simulink model "multirotor_simple_takeoff"  (R2023b)
settings: Solver=VariableStepAuto  StartTime=0.0  StopTime=10.0  RelTol=1e-3
libraries: robotcorelib x1, sensorgpslib x1, uavalgslib x1, uavutilslib x1
settings Model: Creator=rakshan  LastModifiedBy=rakshan
settings DebuggingCC: ParameterPrecisionLossMsg=none

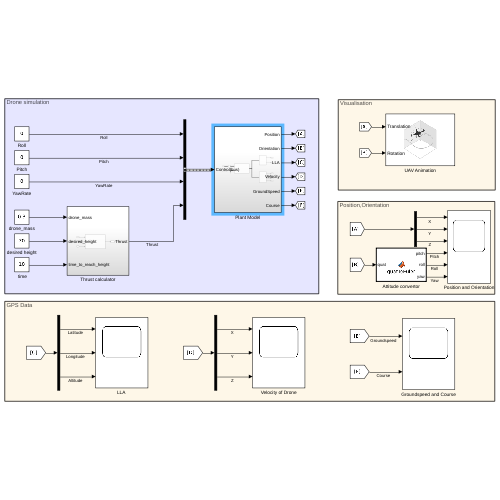
[thumbnail: Simulink's stored preview of the top-level diagram]
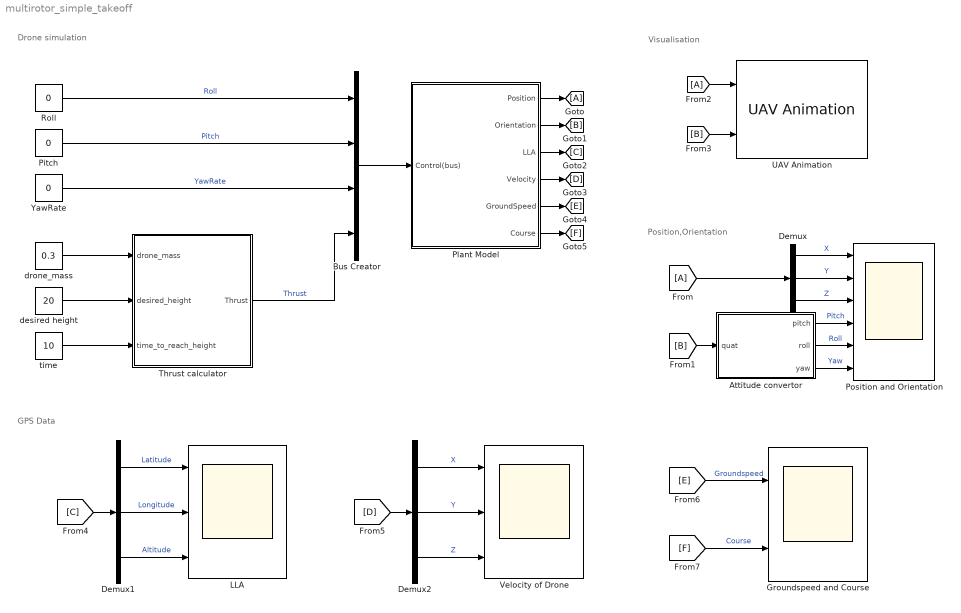
== system multirotor_simple_takeoff ==
  note: GPS Data
  note: Position,Orientation
  note: Visualisation
  note: Drone simulation
  " time" : Constant  Value=10
  Attitude convertor : MATLAB Function  TreatAsAtomicUnit=on
  Bus Creator : BusCreator  Inputs=4  OutDataTypeStr=Bus: uavGuidanceControlBus  NonVirtualBus=on
      settings: InheritFromInputs=off
  Demux : Demux  Outputs=3
  Demux1 : Demux  Outputs=3
  Demux2 : Demux  Outputs=3
  From : From
  From2 : From
  Goto : Goto
  Groundspeed and Course : Scope  NumInputPorts=2
  "LLA " : Scope  NumInputPorts=3
  Pitch : Constant  Value=0  OutDataTypeStr=single
  Plant Model : Subsystem
  Position and Orientation : Scope  NumInputPorts=6
  Roll : Constant  Value=0  OutDataTypeStr=single
  Thrust calculator : Subsystem
  UAV Animation : uavutilslib/UAV Animation  UAVType=Multirotor  UAVSize=3  InertialZDirection=Down  SampleTime=-1
  Velocity of Drone : Scope  NumInputPorts=3
  YawRate : Constant  Value=0  OutDataTypeStr=single
  desired height : Constant  Value=20
  drone_mass : Constant  Value=0.3
  wires:
  Roll/1 -> Bus Creator/1  "Roll"
  Pitch/1 -> Bus Creator/2  "Pitch"
  YawRate/1 -> Bus Creator/3  "YawRate"
  drone_mass/1 -> Thrust calculator/1(drone_mass)
  desired height/1 -> Thrust calculator/2(desired_height)
  " time"/1 -> Thrust calculator/3(time_to_reach_height)
  Thrust calculator/1(Thrust) -> Bus Creator/4  "Thrust"
  Bus Creator/1 -> Plant Model/1(Control(bus))
  Plant Model/1(Position) -> Goto/1
  Plant Model/2(Orientation) -> [B]
  Demux/2 -> Position and Orientation/2  "Y"
  Demux/3 -> Position and Orientation/3  "Z"
  Demux/1 -> Position and Orientation/1  "X"
  Attitude convertor/1(pitch) -> Position and Orientation/4  "Pitch"
  Attitude convertor/2(roll) -> Position and Orientation/5  "Roll"
  Attitude convertor/3(yaw) -> Position and Orientation/6  "Yaw"
  From/1 -> Demux/1
  [B] -> Attitude convertor/1(quat)
  Plant Model/3(LLA) -> [C]
  Plant Model/4(Velocity) -> [D]
  Plant Model/5(GroundSpeed) -> [E]
  Plant Model/6(Course) -> [F]
  From2/1 -> UAV Animation/1
  [B] -> UAV Animation/2
  Demux1/2 -> "LLA "/2  "Longitude"
  Demux1/1 -> "LLA "/1  "Latitude"
  Demux1/3 -> "LLA "/3  "Altitude"
  [C] -> Demux1/1
  Demux2/2 -> Velocity of Drone/2  "Y"
  Demux2/3 -> Velocity of Drone/3  "Z"
  [D] -> Demux2/1
  Demux2/1 -> Velocity of Drone/1  "X"
  [E] -> Groundspeed and Course/1  "Groundspeed"
  [F] -> Groundspeed and Course/2  "Course"

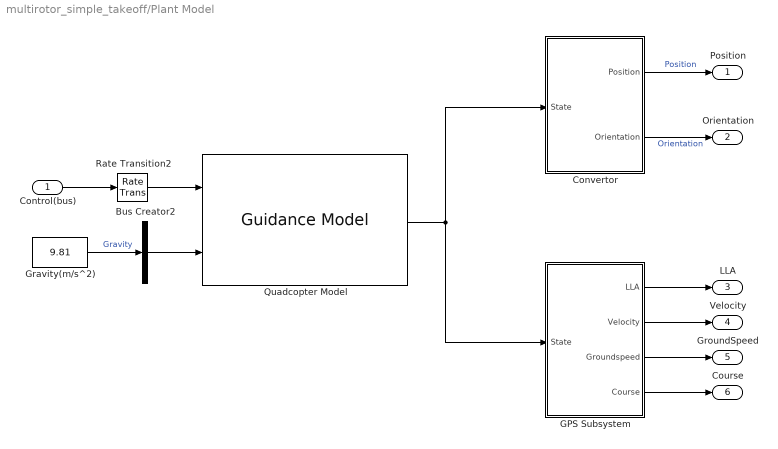
== system multirotor_simple_takeoff/Plant Model ==
  Control(bus) : Inport
  Bus Creator2 : BusCreator  Inputs=1  OutDataTypeStr=Bus: uavGuidanceEnvironmentBus  NonVirtualBus=on
  Convertor : Subsystem
  GPS Subsystem : Subsystem
  Gravity(m/s^2) : Constant  Value=9.81  OutDataTypeStr=single
  Quadcopter Model : uavalgslib/Guidance Model  ModelType=MultirotorGuidance  SpecifiedDataType=single  SimulateUsing=Code generation  InitialWorldPositionMultirotor=[0; 0; 0]  InitialWorldVelocityMultirotor=[0; 0; 0]  InitialEulerZYXMultirotor=[0; 0; 0]  InitialBodyAngularRateRPYMultirotor=[0; 0; 0]  InitialThrustMultirotor=0  InitialNorthFixedWing=0  InitialEastFixedWing=0  InitialHeightFixedWing=0  InitialAirSpeedFixedWing=0  InitialHeadingAngleFixedWing=0  InitialFlightPathAngleFixedWing=0  InitialRollAngleFixedWing=0  InitialRollAngleRateFixedWing=0  PDRollMultirotor=[3402.97,116.67]  PDPitchMultirotor=[3402.97, 116.67]  PYawRateMultirotor=1950  PThrustMultirotor=3900  MassMultirotor=0.3  PHeightFixedWing=3.9  PHeadingAngleFixedWing=3.9  PFlightPathAngleFixedWing=39  PDRollFixedWing=[3402.97, 116.67]  PAirSpeedFixedWing=1  FlightPathAngleLimitsFixedWing=[-pi/2, pi/2]  StateBusName='uavGuidanceStateBus'  ControlBusName='uavGuidanceControlBus'  EnvironmentBusName='uavGuidanceEnvironmentBus'  DataType=single
  Rate Transition2 : RateTransition
  Position : Outport
  Orientation : Outport  Port=2
  LLA : Outport  Port=3
  Velocity : Outport  Port=4
  GroundSpeed : Outport  Port=5
  Course : Outport  Port=6
  wires:
  Rate Transition2/1 -> Quadcopter Model/1
  Quadcopter Model/1 -> Convertor/1(State), GPS Subsystem/1(State)
  Bus Creator2/1 -> Quadcopter Model/2
  Control(bus)/1 -> Rate Transition2/1
  Gravity(m/s^2)/1 -> Bus Creator2/1  "Gravity"
  Convertor/1(Position) -> Position/1  "Position"
  Convertor/2(Orientation) -> Orientation/1  "Orientation"
  GPS Subsystem/1(LLA) -> LLA/1
  GPS Subsystem/2(Velocity) -> Velocity/1
  GPS Subsystem/3(Groundspeed) -> GroundSpeed/1
  GPS Subsystem/4(Course) -> Course/1

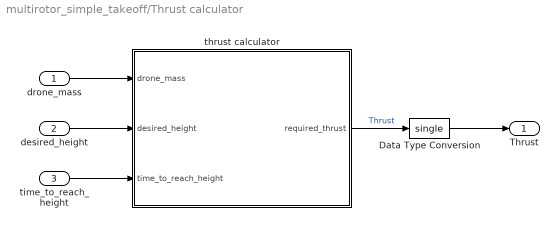
== system multirotor_simple_takeoff/Thrust calculator ==
  drone_mass : Inport
  desired_height : Inport  Port=2
  time_to_reach_height : Inport  Port=3
  Data Type Conversion : DataTypeConversion  OutDataTypeStr=single  SaturateOnIntegerOverflow=off  RndMeth=Floor
  thrust calculator : MATLAB Function  TreatAsAtomicUnit=on
  Thrust : Outport
  wires:
  Data Type Conversion/1 -> Thrust/1
  time_to_reach_height/1 -> thrust calculator/3(time_to_reach_height)
  drone_mass/1 -> thrust calculator/1(drone_mass)
  thrust calculator/1(required_thrust) -> Data Type Conversion/1  "Thrust"
  desired_height/1 -> thrust calculator/2(desired_height)

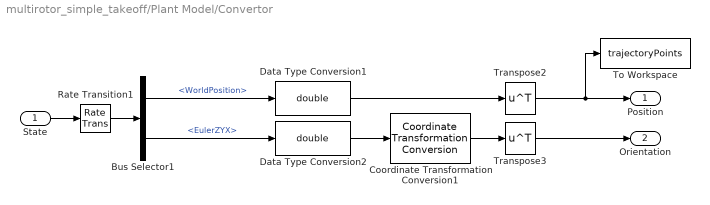
== system multirotor_simple_takeoff/Plant Model/Convertor ==
  State : Inport
  Bus Selector1 : BusSelector  OutputSignals=WorldPosition,EulerZYX
  Coordinate Transformation Conversion1 : robotcorelib/Coordinate Transformation Conversion  InputRepresentation=Euler Angles  InputEulerSequence=ZYX  ShowTrVecInputPort=on  OutputRepresentation=Quaternion  OutputEulerSequence=ZYX  ShowTrVecOutputPort=on  SimulateUsing=Code generation
  Data Type Conversion1 : DataTypeConversion  OutDataTypeStr=double  SaturateOnIntegerOverflow=off  RndMeth=Floor
  Data Type Conversion2 : DataTypeConversion  OutDataTypeStr=double  SaturateOnIntegerOverflow=off  RndMeth=Floor
  Rate Transition1 : RateTransition
  To Workspace : ToWorkspace  VariableName=trajectoryPoints  SampleTime=-1
  Transpose2 : Math  Operator=transpose
  Transpose3 : Math  Operator=transpose
  Position : Outport
  Orientation : Outport  Port=2
  wires:
  State/1 -> Rate Transition1/1
  Transpose2/1 -> To Workspace/1, Position/1
  Bus Selector1/1 -> Data Type Conversion1/1  "<WorldPosition>"
  Data Type Conversion2/1 -> Coordinate Transformation Conversion1/1
  Bus Selector1/2 -> Data Type Conversion2/1  "<EulerZYX>"
  Coordinate Transformation Conversion1/1 -> Transpose3/1
  Transpose3/1 -> Orientation/1
  Data Type Conversion1/1 -> Transpose2/1
  Rate Transition1/1 -> Bus Selector1/1

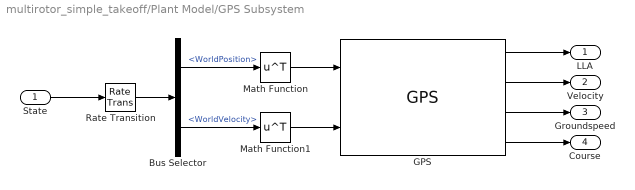
== system multirotor_simple_takeoff/Plant Model/GPS Subsystem ==
  State : Inport
  Bus Selector : BusSelector  OutputSignals=WorldPosition,WorldVelocity
  GPS : sensorgpslib/GPS  DispRefFrame=NED  PositionInputFormat=Geodetic  ReferenceLocation=[ 0, 0, 0 ]  HorizontalPositionAccuracy=1.6  VerticalPositionAccuracy=3  VelocityAccuracy=0.1  DecayFactor=0.999  SeedDouble=63  SimulateUsing=Interpreted execution
      settings: LibrarySourceBlock=uavsimlib/GPS
  Math Function : Math  Operator=transpose  SignedPower=on  RndMeth=Zero
  Math Function1 : Math  Operator=transpose  SignedPower=on  RndMeth=Zero
  Rate Transition : RateTransition  OutPortSampleTime=0.01
  LLA : Outport
  Velocity : Outport  Port=2
  Groundspeed : Outport  Port=3
  Course : Outport  Port=4
  wires:
  Math Function/1 -> GPS/1
  Rate Transition/1 -> Bus Selector/1
  GPS/2 -> Velocity/1
  Math Function1/1 -> GPS/2
  Bus Selector/2 -> Math Function1/1  "<WorldVelocity>"
  GPS/4 -> Course/1
  GPS/1 -> LLA/1
  State/1 -> Rate Transition/1
  Bus Selector/1 -> Math Function/1  "<WorldPosition>"
  GPS/3 -> Groundspeed/1

== matlab function multirotor_simple_takeoff/Thrust calculator/thrust calculator ==
  data: drone_mass input; required_thrust output; desired_height input; time_to_reach_height input
function required_thrust = calculate_thrust(drone_mass, desired_height, time_to_reach_height)
    % Constants
    g = 9.81;  % gravitational acceleration (m/s^2)
    
    % Calculate the required acceleration (assuming uniform acceleration)
    required_acceleration = 2 * desired_height / (time_to_reach_height ^ 2);
    
    % Total required thrust (mass * (g + required_acceleration))
    required_thrust = drone_mass * (g + required_acceleration);
end

== matlab function multirotor_simple_takeoff/Attitude convertor ==
  data: quat input; pitch output; roll output; yaw output
function [pitch, roll, yaw] = quatToEuler(quat)
    % Ensure the quaternion is a unit quaternion
    quat = quat / norm(quat);

    % Extract the components of the quaternion
    w = quat(1);
    x = quat(2);
    y = quat(3);
    z = quat(4);

    % Compute the roll (x-axis rotation)
    sinr_cosp = 2 * (w * x + y * z);
    cosr_cosp = 1 - 2 * (x * x + y * y);
    roll = atan2(sinr_cosp, cosr_cosp);

    % Compute the pitch (y-axis rotation)
    sinp = 2 * (w * y - z * x);
    if abs(sinp) >= 1
        pitch = sign(sinp) * pi / 2; % Use 90 degrees if out of range
    else
        pitch = asin(sinp);
    end

    % Compute the yaw (z-axis rotation)
    siny_cosp = 2 * (w * z + x * y);
    cosy_cosp = 1 - 2 * (y * y + z * z);
    yaw = atan2(siny_cosp, cosy_cosp);
end
